simulink model "task7"  (R2023a)
settings: Solver=VariableStepAuto  StartTime=0.0  StopTime=100  RelTol=1e-3
undefined symbols (not defined in the file or in its folder): DisplayEllipses
settings Model: SimulationMode=accelerator  Creator=LENOVO  LastModifiedBy=LENOVO

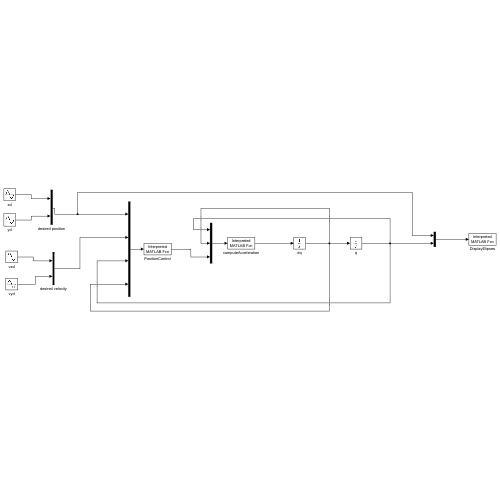
[thumbnail: Simulink's stored preview of the top-level diagram]
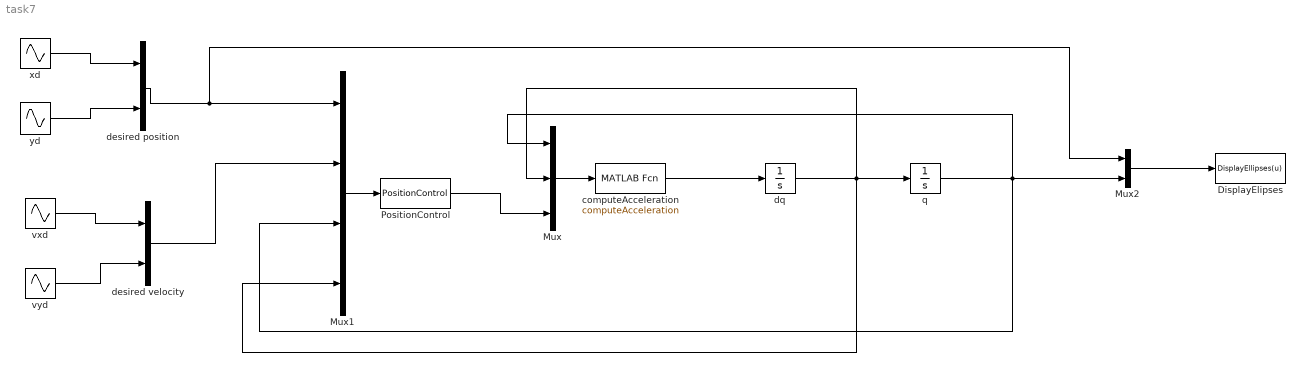
== system task7 ==
  DisplayElipses : MATLABFcn  MATLABFcn=DisplayEllipses(u)  OutputDimensions=0
  Mux : Mux  Inputs=3
  Mux1 : Mux
  Mux2 : Mux  Inputs=2
  PositionControl : MATLABFcn  MATLABFcn=PositionControl  OutputDimensions=2
  computeAcceleration : MATLABFcn  MATLABFcn=computeAcceleration  OutputDimensions=2  Output1D=off
  desired position : Mux  Inputs=2
  desired velocity : Mux  Inputs=2
  dq : Integrator  InitialCondition=[0; 0]
  q : Integrator  InitialCondition=[pi/2; pi/4]
  vxd : Sin  Amplitude=0.15*2/3*pi  Frequency=1/3*2*pi  Phase=90  SampleTime=0
  vyd : Sin  Amplitude=-0.1*2/3*pi  Frequency=2*1/3*pi  SampleTime=0
  xd : Sin  Amplitude=0.15  Bias=0.15  Frequency=1/3*2*pi  SampleTime=0
  yd : Sin  Amplitude=0.1  Bias=0.2  Frequency=1/3*2*pi  Phase=90  SampleTime=0
  wires:
  dq/1 -> Mux1/4, Mux/2, q/1
  q/1 -> Mux1/3, Mux/1, Mux2/2
  Mux/1 -> computeAcceleration/1
  computeAcceleration/1 -> dq/1
  xd/1 -> desired position/1
  yd/1 -> desired position/2
  vxd/1 -> desired velocity/1
  vyd/1 -> desired velocity/2
  desired position/1 -> Mux2/1, Mux1/1
  desired velocity/1 -> Mux1/2
  Mux1/1 -> PositionControl/1
  PositionControl/1 -> Mux/3
  Mux2/1 -> DisplayElipses/1
